simulink model "ACC_Discrete"  (R2013b)
settings: Solver=ode45  StartTime=0.0  StopTime=10.0  RelTol=1e-3
undefined symbols (not defined in the file): DiscIntNeverNeededParam
libraries: simulink x2
settings Model: Creator=user  LastModifiedBy=user
settings DataIOCC: SignalLoggingSaveFormat=ModelDataLogs
settings DebuggingCC: UnderspecifiedInitializationDetection=Simplified  MultiTaskDSMMsg=warning  MultiTaskCondExecSysMsg=none  StrictBusMsg=None
settings RTWCC: IncludeERTFirstTime=on
settings GRTTargetCC: CodeReplacementLibrary=None  CPPClassGenCompliant=on

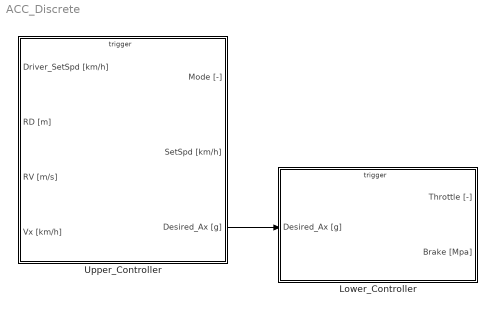
== system ACC_Discrete ==
  Lower_Controller : Subsystem
  Upper_Controller : Subsystem
  wires:
  Upper_Controller/3(Desired_Ax [g]) -> Lower_Controller/1(Desired_Ax [g])

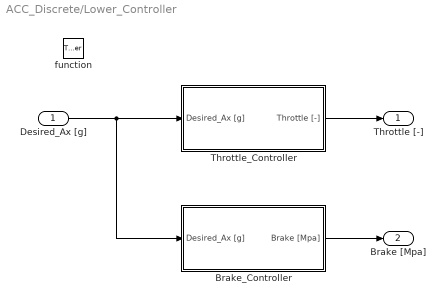
== system ACC_Discrete/Lower_Controller ==
  Desired_Ax [g] : Inport
  function : TriggerPort  TriggerType=function-call
  Brake_Controller : Subsystem
  Throttle_Controller : Subsystem
  Throttle [-] : Outport
  Brake [Mpa] : Outport  Port=2
  wires:
  Desired_Ax [g]/1 -> Brake_Controller/1(Desired_Ax [g]), Throttle_Controller/1(Desired_Ax [g])
  Throttle_Controller/1(Throttle [-]) -> Throttle [-]/1
  Brake_Controller/1(Brake [Mpa]) -> Brake [Mpa]/1

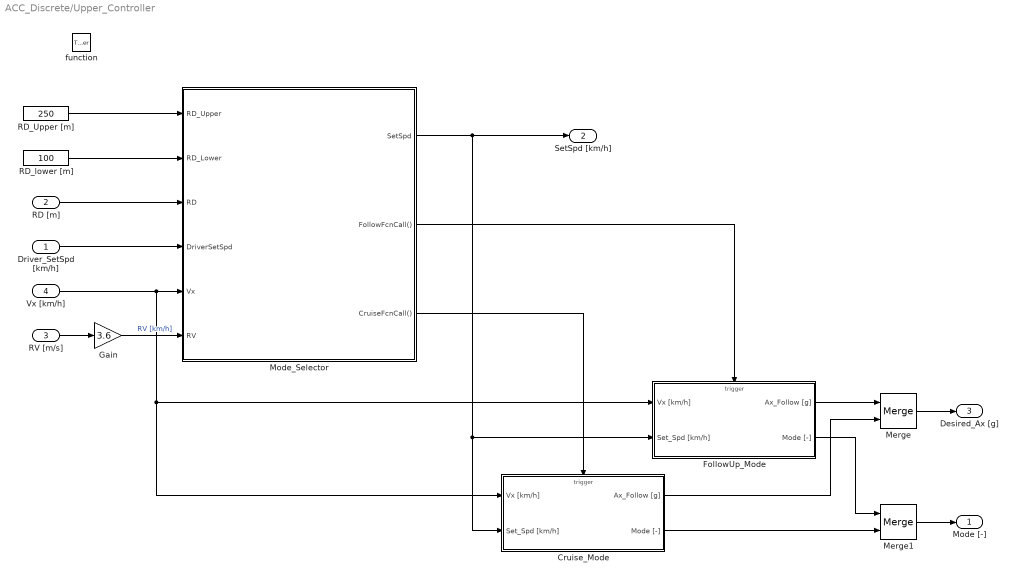
== system ACC_Discrete/Upper_Controller ==
  Driver_SetSpd [km/h] : Inport
  RD [m] : Inport  Port=2
  RV [m/s] : Inport  Port=3
  Vx [km/h] : Inport  Port=4
  function : TriggerPort  TriggerType=function-call
  Cruise_Mode : Subsystem  TreatAsAtomicUnit=on
  FollowUp_Mode : Subsystem  TreatAsAtomicUnit=on
  Gain : Gain  Gain=3.6
  Merge : Merge
  Merge1 : Merge
  Mode_Selector : Stateflow chart  TreatAsAtomicUnit=on
  RD_Upper [m] : Constant  Value=250
  RD_lower [m] : Constant  Value=100
  Mode [-] : Outport
  SetSpd [km/h] : Outport  Port=2
  Desired_Ax [g] : Outport  Port=3
  wires:
  RD_lower [m]/1 -> Mode_Selector/2(RD_Lower)
  RD_Upper [m]/1 -> Mode_Selector/1(RD_Upper)
  Driver_SetSpd [km/h]/1 -> Mode_Selector/4(DriverSetSpd)
  RD [m]/1 -> Mode_Selector/3(RD)
  Vx [km/h]/1 -> FollowUp_Mode/1(Vx [km/h]), Cruise_Mode/1(Vx [km/h]), Mode_Selector/5(Vx)
  RV [m/s]/1 -> Gain/1
  Gain/1 -> Mode_Selector/6(RV)  "RV [km/h]"
  Cruise_Mode/1(Ax_Follow [g]) -> Merge/2
  FollowUp_Mode/2(Mode [-]) -> Merge1/1
  Cruise_Mode/2(Mode [-]) -> Merge1/2
  Merge/1 -> Desired_Ax [g]/1
  Merge1/1 -> Mode [-]/1
  Mode_Selector/1(SetSpd) -> Cruise_Mode/2(Set_Spd [km/h]), FollowUp_Mode/2(Set_Spd [km/h]), SetSpd [km/h]/1
  Mode_Selector/2(FollowFcnCall()) -> FollowUp_Mode/Trigger
  Mode_Selector/3(CruiseFcnCall()) -> Cruise_Mode/Trigger
  FollowUp_Mode/1(Ax_Follow [g]) -> Merge/1

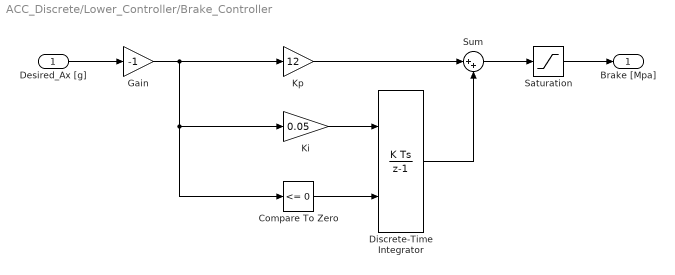
== system ACC_Discrete/Lower_Controller/Brake_Controller ==
  Desired_Ax [g] : Inport
  Compare To Zero : simulink/Logic and Bit Operations/Compare To Zero  relop=<=  OutDataTypeStr=boolean
  Discrete-Time Integrator : DiscreteIntegrator  ExternalReset=rising  ICPrevOutput=DiscIntNeverNeededParam  ICPrevScaledInput=DiscIntNeverNeededParam
  Gain : Gain  Gain=-1
  Ki : Gain  Gain=0.05
  Kp : Gain  Gain=12
  Saturation : Saturate  UpperLimit=6  LowerLimit=0
  Sum : Sum  Inputs=|++
  Brake [Mpa] : Outport
  wires:
  Sum/1 -> Saturation/1
  Saturation/1 -> Brake [Mpa]/1
  Desired_Ax [g]/1 -> Gain/1
  Kp/1 -> Sum/1
  Ki/1 -> Discrete-Time Integrator/1
  Discrete-Time Integrator/1 -> Sum/2
  Gain/1 -> Compare To Zero/1, Ki/1, Kp/1
  Compare To Zero/1 -> Discrete-Time Integrator/2

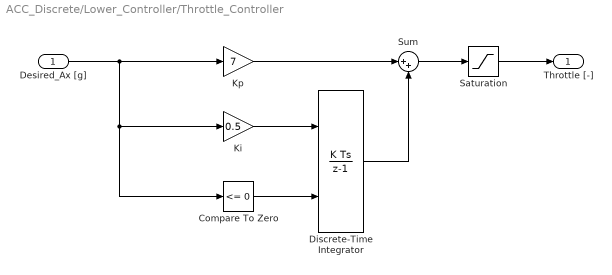
== system ACC_Discrete/Lower_Controller/Throttle_Controller ==
  Desired_Ax [g] : Inport
  Compare To Zero : simulink/Logic and Bit Operations/Compare To Zero  relop=<=  OutDataTypeStr=boolean
  Discrete-Time Integrator : DiscreteIntegrator  ExternalReset=rising  ICPrevOutput=DiscIntNeverNeededParam  ICPrevScaledInput=DiscIntNeverNeededParam
  Ki : Gain  Gain=0.5
  Kp : Gain  Gain=7
  Saturation : Saturate  UpperLimit=0.7  LowerLimit=0
  Sum : Sum  Inputs=|++
  Throttle [-] : Outport
  wires:
  Sum/1 -> Saturation/1
  Saturation/1 -> Throttle [-]/1
  Desired_Ax [g]/1 -> Compare To Zero/1, Ki/1, Kp/1
  Kp/1 -> Sum/1
  Ki/1 -> Discrete-Time Integrator/1
  Compare To Zero/1 -> Discrete-Time Integrator/2
  Discrete-Time Integrator/1 -> Sum/2

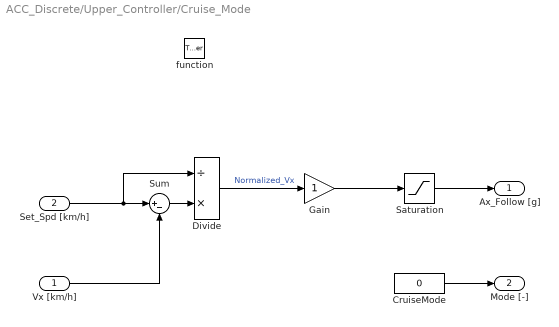
== system ACC_Discrete/Upper_Controller/Cruise_Mode ==
  Vx [km/h] : Inport
  Set_Spd [km/h] : Inport  Port=2
  function : TriggerPort  TriggerType=function-call
  CruiseMode : Constant  Value=0
  Divide : Product  Inputs=/*
  Gain : Gain
  Saturation : Saturate  UpperLimit=0.3  LowerLimit=-0.3
  Sum : Sum  Inputs=|+-
  Ax_Follow [g] : Outport
  Mode [-] : Outport  Port=2
  wires:
  Set_Spd [km/h]/1 -> Divide/1, Sum/1
  Vx [km/h]/1 -> Sum/2
  Sum/1 -> Divide/2
  Divide/1 -> Gain/1  "Normalized_Vx"
  Gain/1 -> Saturation/1
  Saturation/1 -> Ax_Follow [g]/1
  CruiseMode/1 -> Mode [-]/1

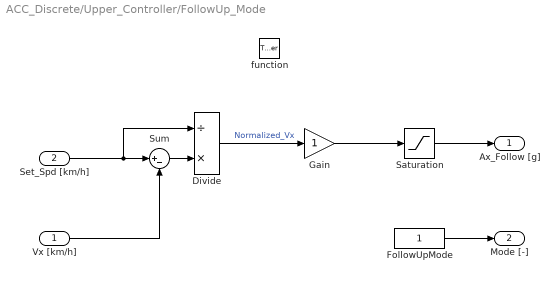
== system ACC_Discrete/Upper_Controller/FollowUp_Mode ==
  Vx [km/h] : Inport
  Set_Spd [km/h] : Inport  Port=2
  function : TriggerPort  TriggerType=function-call
  Divide : Product  Inputs=/*
  FollowUpMode : Constant
  Gain : Gain
  Saturation : Saturate  UpperLimit=0.4  LowerLimit=-0.4
  Sum : Sum  Inputs=|+-
  Ax_Follow [g] : Outport
  Mode [-] : Outport  Port=2
  wires:
  Set_Spd [km/h]/1 -> Divide/1, Sum/1
  Vx [km/h]/1 -> Sum/2
  Sum/1 -> Divide/2
  Divide/1 -> Gain/1  "Normalized_Vx"
  Gain/1 -> Saturation/1
  Saturation/1 -> Ax_Follow [g]/1
  FollowUpMode/1 -> Mode [-]/1

== stateflow chart ACC_Discrete/Upper_Controller/Mode_Selector ==
  state Cruise_Mode
    du, en : TVSpd = RV+Vx;
    du : send(CruiseFcnCall)
    du : SetSpd = DriverSetSpd;
  state FollowUp_Mode
    du, en : TVSpd = RV+Vx;
    du : send(FollowFcnCall)
    du : SetSpd = TVSpd;
  (default) -> Cruise_Mode
  Cruise_Mode -> FollowUp_Mode : [(RD<=RD_Lower) & (DriverSetSpd >= TVSpd)]
  FollowUp_Mode -> Cruise_Mode : [(RD>RD_Upper) | (DriverSetSpd < TVSpd)]
  data: RD_Upper input; RD_Lower input; RD input; DriverSetSpd input; SetSpd output; Vx input; RV input; TVSpd local
  events: FollowFcnCall output FUNCTION_CALL_EVENT; CruiseFcnCall output FUNCTION_CALL_EVENT
